simulink model "QPSK-SImulink"  (R2020b)
settings: Solver=VariableStepAuto  StartTime=0.0  StopTime=10.0  RelTol=1e-3
libraries: commdigbbndpm3 x2, commchan3 x1, commsink2 x1, commrandsrc2 x1
settings Model: Creator=MRUNMAYEE J. MORE  LastModifiedBy=MRUNMAYEE J. MORE

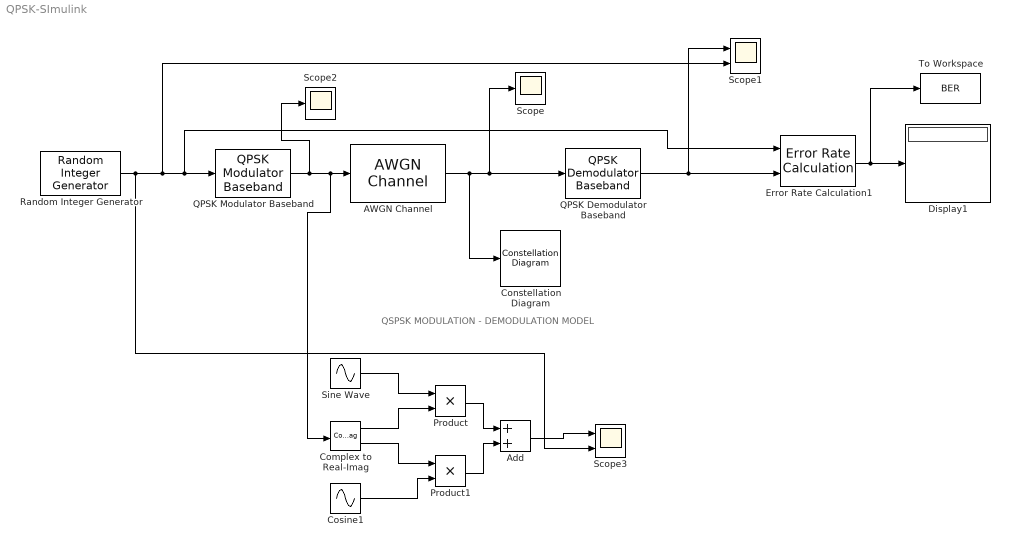
== system QPSK-SImulink ==
  note: QSPSK MODULATION - DEMODULATION MODEL
  AWGN Channel : commchan3/AWGN Channel  InputProcessing=Columns as channels (frame based)  seed=67  noiseMode="Signal to noise ratio  (Eb/No)"  EbNodB=0  EsNodB=10  SNRdB=10  bitsPerSym=2  Ps=1  Tsym=1  variance=1
  Add : Sum
  Complex to Real-Imag : ComplexToRealImag
  Constellation Diagram : ConstellationDiagram
  Cosine1 : Sin  Frequency=8*pi  Phase=pi/2  SampleTime=0.001
  Display1 : Display
  Error Rate Calculation1 : commsink2/Error Rate Calculation  N=0  st_delay=0  cp_mode=Entire frame  subframe=[]  PMode=Port  WsName=ErrorVec  RsMode2=off  stop=on  numErr=1e3  maxBits=1e6
  Product : Product
  Product1 : Product
  QPSK Demodulator Baseband : commdigbbndpm3/QPSK Demodulator Baseband  OutType=Integer  DecType=Hard decision  VarSource=Dialog  Variance=1  Dec=Gray  Ph=pi/2  outDtype1=Inherit via internal rule  outDtype2=Inherit via internal rule  derotateFactorWordLen=16  derotateFactorDataTypeStr=Inherit: Same word length as input  derotateFactorLastDataTypeStr=Inherit: Same word length as input
  QPSK Modulator Baseband : commdigbbndpm3/QPSK Modulator Baseband  InType=Integer  Enc=Gray  Ph=pi/4  outDtype=double  outWordLen=16  outUDDataType=sfix(16)  outFracLenMode=Best precision  outFracLen=15  outDataTypeStr=double  outLastDataTypeStr=double
  Random Integer Generator : commrandsrc2/Random Integer Generator  mul=4  seed=67  Ts=1  frameBased=on  sampPerFrame=1  orient=off  outDataType=double
      settings: SourceProductBaseCode=CM
  Scope : Scope
  Scope1 : Scope  NumInputPorts=2
  Scope2 : Scope
  Scope3 : Scope  NumInputPorts=2
  Sine Wave : Sin  Frequency=8*pi  SampleTime=0.001
  To Workspace : ToWorkspace  VariableName=BER  SampleTime=-1
      settings: MaxDataPoints=1
  wires:
  QPSK Demodulator Baseband/1 -> Error Rate Calculation1/2, Scope1/1
  AWGN Channel/1 -> Scope/1, QPSK Demodulator Baseband/1, Constellation Diagram/1
  QPSK Modulator Baseband/1 -> Scope2/1, Complex to Real-Imag/1, AWGN Channel/1
  Random Integer Generator/1 -> Scope1/2, Error Rate Calculation1/1, QPSK Modulator Baseband/1, Scope3/2
  Complex to Real-Imag/1 -> Product/2
  Complex to Real-Imag/2 -> Product1/1
  Sine Wave/1 -> Product/1
  Cosine1/1 -> Product1/2
  Product/1 -> Add/1
  Product1/1 -> Add/2
  Add/1 -> Scope3/1
  Error Rate Calculation1/1 -> Display1/1, To Workspace/1
